simulink model "sdbe_8pac_11"  (R2012b)
settings: Solver=VariableStepDiscrete  SolverMode=SingleTasking  StartTime=0.0  StopTime=10000  RelTol=1e-3
PreLoadFcn:
  | counter_vals
undefined symbols (not defined in the file or in its folder): sfp
libraries: xbsIndex_r4 x9355, casper_library_misc x39, casper_library_delays x27, dspsigops x16, xps_library x10, r2dbe_vdif_lib x4, r2dbe_adc_lib x3, simulink x1
(part 31 of 79)

== system sdbe_8pac_11/valid_eof_snap_0x/bram ==
  addr : Inport
  data_in : Inport  Port=2
  we : Inport  Port=3
  calc_add : Subsystem  mask{data_width=16, addr_width=14, sample_rate=sample_rate}
      mask prompts: data_width "data width"; addr_width "address width"; sample_rate "sample rate"
  convert_addr : xbsIndex_r4/Convert  gui_display_data_type=Fixed-point  arith_type=Unsigned  n_bits=addr_width  bin_pt=0  float_type=Single  exp_bits=8  fraction_bits=24  quantization=Truncate  overflow=Wrap  en=off  latency=0  dbl_ovrd=off  pipeline=off  block_type=convert
      settings: xl_area=[0, 0, 0, 0, 0, 0, 0]
  convert_din1 : xbsIndex_r4/Convert  gui_display_data_type=Fixed-point  arith_type=Unsigned  n_bits=16  bin_pt=0  float_type=Single  exp_bits=8  fraction_bits=24  quantization=Truncate  overflow=Wrap  en=off  latency=0  dbl_ovrd=off  pipeline=off  block_type=convert
      settings: xl_area=[0, 0, 0, 0, 0, 0, 0]
  convert_we : xbsIndex_r4/Convert  gui_display_data_type=Fixed-point  arith_type=Unsigned  n_bits=1  bin_pt=0  float_type=Single  exp_bits=8  fraction_bits=24  quantization=Truncate  overflow=Wrap  en=off  latency=0  dbl_ovrd=off  pipeline=off  block_type=convert
      settings: xl_area=[0, 0, 0, 0, 0, 0, 0]
  mem : Subsystem
  munge_in : Subsystem  AncestorBlock=casper_library_flow_control/munge  mask(munge){divisions=1, div_size=16, order=[0], arith_type_out=Unsigned, bin_pt_out=0}
      mask prompts: divisions "Number of divisions"; div_size "Division size (bits)"; order "Division packing order"; arith_type_out "Output arithmetic type"; bin_pt_out "Output binary point"
      mask help: Splits an input bus into the specified number of divisions and then recombines them in the order specified (most significant division = 0,least = number divisions-1)
      mask init:
      | munge_init(gcb, ...
      |     'divisions', divisions, ...
      |     'div_size', div_size, ...
      |     'order', order, ...
      |     'arith_type_out', arith_type_out, ...
      |     'bin_pt_out', bin_pt_out);
      settings: AttributesFormatString=|
      | split:16
      | join:0
      | Unsigned [16,0]
      mask TypeOptions arith_type_out: Unsigned | Signed  (2's comp) | Floating-point
  munge_out : Subsystem  AncestorBlock=casper_library_flow_control/munge  mask(munge){divisions=1, div_size=16, order=[0], arith_type_out=Unsigned, bin_pt_out=0}
      mask prompts: divisions "Number of divisions"; div_size "Division size (bits)"; order "Division packing order"; arith_type_out "Output arithmetic type"; bin_pt_out "Output binary point"
      mask help: Splits an input bus into the specified number of divisions and then recombines them in the order specified (most significant division = 0,least = number divisions-1)
      mask init:
      | munge_init(gcb, ...
      |     'divisions', divisions, ...
      |     'div_size', div_size, ...
      |     'order', order, ...
      |     'arith_type_out', arith_type_out, ...
      |     'bin_pt_out', bin_pt_out);
      settings: AttributesFormatString=|
      | split:16
      | join:0
      | Unsigned [16,0]
      mask TypeOptions arith_type_out: Unsigned | Signed  (2's comp) | Floating-point
  sdbe_8pac_11_valid_eof_snap_0x_bram_addr : xbsIndex_r4/Gateway Out  inherit_from_input=off  hdl_port=on  timing_constraint=None  locs_specified=off  LOCs={'A5','B9','A9','C1','A3','G6','E9','A6','A7','A8','B8','B1','B3','D9','B5','B4','B6','C2'}  UseAsDAC=off  DACChannel='1'  block_type=gatewayout
      settings: infoedit="Gateway out block.  Converts Xilinx fixed point inputs into ouputs of type Simulink integer, double, or fixed point.<P><P>Hardware notes:  In hardware these blocks become top level output ports or are discarded, depending on how they are configured."  xl_area=[0, 0, 0, 0, 0, 0, 0]  sginterface={'Nallatech'=>{'xdspkit'=>{'non_memory_mapped_port'=>'uprev_Shared_BRAM_addr'}},'Xilinx'=>{'jtaghwcosim'=>{'non_memory_mapped_port'=>'uprev_Shared_BRAM_addr'},'xdspkit'=>{'non_memory_mapped_port'=>'uprev_Shared_BRAM_addr'}}}
  sdbe_8pac_11_valid_eof_snap_0x_bram_data_in : xbsIndex_r4/Gateway Out  inherit_from_input=off  hdl_port=on  timing_constraint=None  locs_specified=off  LOCs={'B21','B22','A22','B23','B19','C19','A20','A21','A23','B24','A24','A25','E18','D18','C18','B18'}  UseAsDAC=off  DACChannel='1'  block_type=gatewayout
      settings: infoedit="Gateway out block.  Converts Xilinx fixed point inputs into ouputs of type Simulink integer, double, or fixed point.<P><P>Hardware notes:  In hardware these blocks become top level output ports or are discarded, depending on how they are configured."  xl_area=[0, 0, 0, 0, 0, 0, 0]  sginterface={'Nallatech'=>{'xdspkit'=>{'non_memory_mapped_port'=>'uprev_Shared_BRAM_data_in'}},'Xilinx'=>{'jtaghwcosim'=>{'non_memory_mapped_port'=>'uprev_Shared_BRAM_data_in'},'xdspkit'=>{'non_memory_mapped_port'=>'uprev_Shared_BRAM_data_in'}}}
  sdbe_8pac_11_valid_eof_snap_0x_bram_data_out : xbsIndex_r4/Gateway In  gui_display_data_type=Fixed-point  arith_type=Unsigned  n_bits=16  bin_pt=0  preci_type=Single  exp_width=8  frac_width=24  quantization=Truncate  overflow=Wrap  period=sample_rate  dbl_ovrd=off  timing_constraint=None  locs_specified=off  LOCs={}  UseAsADC=off  ADCChannel='1'  inherit_from_input=off  hdl_port=on  block_type=gatewayin
      settings: xl_area=[0, 0, 0, 0, 0, 0, 0]
  sdbe_8pac_11_valid_eof_snap_0x_bram_we : xbsIndex_r4/Gateway Out  inherit_from_input=off  hdl_port=on  timing_constraint=None  locs_specified=off  LOCs={'A14'}  UseAsDAC=off  DACChannel='1'  block_type=gatewayout
      settings: infoedit="Gateway out block.  Converts Xilinx fixed point inputs into ouputs of type Simulink integer, double, or fixed point.<P><P>Hardware notes:  In hardware these blocks become top level output ports or are discarded, depending on how they are configured."  xl_area=[0, 0, 0, 0, 0, 0, 0]
  data_out : Outport
  wires:
  convert_addr/1 -> sdbe_8pac_11_valid_eof_snap_0x_bram_addr/1
  convert_din1/1 -> sdbe_8pac_11_valid_eof_snap_0x_bram_data_in/1
  data_in/1 -> munge_in/1(din)
  calc_add/1(out) -> convert_addr/1
  sdbe_8pac_11_valid_eof_snap_0x_bram_we/1 -> mem/3(In3)
  sdbe_8pac_11_valid_eof_snap_0x_bram_data_in/1 -> mem/2(In2)
  sdbe_8pac_11_valid_eof_snap_0x_bram_addr/1 -> mem/1(In1)
  convert_we/1 -> sdbe_8pac_11_valid_eof_snap_0x_bram_we/1
  sdbe_8pac_11_valid_eof_snap_0x_bram_data_out/1 -> munge_out/1(din)
  mem/1(Out1) -> sdbe_8pac_11_valid_eof_snap_0x_bram_data_out/1
  addr/1 -> calc_add/1(in)
  we/1 -> convert_we/1
  munge_out/1(dout) -> data_out/1
  munge_in/1(dout) -> convert_din1/1

== system sdbe_8pac_11/valid_eof_snap_0x/ctrl ==
  sim_1 : Inport
  io_delay : xbsIndex_r4/Delay  rst=off  infoeditControl=Selection of Reset will increase slice count due to use of real FFs and instead of SRLs  en=off  latency=0  dbl_ovrd=off  reg_retiming=on  block_type=delay
  reint1 : xbsIndex_r4/Reinterpret  force_arith_type=on  arith_type=Unsigned  force_bin_pt=on  bin_pt=0  block_type=reinterpret
  sdbe_8pac_11_valid_eof_snap_0x_ctrl_user_data_out : xbsIndex_r4/Gateway In  gui_display_data_type=Fixed-point  arith_type=Unsigned  n_bits=32  bin_pt=0  preci_type=Single  exp_width=8  frac_width=24  quantization="Round  (unbiased: +/- Inf)"  overflow=Saturate  period=1  dbl_ovrd=off  timing_constraint=None  locs_specified=off  LOCs={}  UseAsADC=off  ADCChannel='1'  inherit_from_input=off  hdl_port=on  block_type=gatewayin
  slice_reg : xbsIndex_r4/Slice  nbits=32  boolean_output=off  mode=Lower Bit Location + Width  bit1=0  base1=MSB of Input  bit0=0  base0=LSB of Input  dbl_ovrd=off  block_type=slice
  in_reg : Outport
  wires:
  sdbe_8pac_11_valid_eof_snap_0x_ctrl_user_data_out/1 -> io_delay/1
  sim_1/1 -> sdbe_8pac_11_valid_eof_snap_0x_ctrl_user_data_out/1
  io_delay/1 -> slice_reg/1
  slice_reg/1 -> reint1/1
  reint1/1 -> in_reg/1

== system sdbe_8pac_11/valid_eof_snap_0x/status ==
  out_reg : Inport
  assert_reg : xbsIndex_r4/Assert  assert_type=on  type_source=Explicitly  gui_display_data_type=Fixed-point  arith_type=Unsigned  n_bits=32  bin_pt=0  preci_type=Single  exp_width=8  frac_width=24  assert_rate=off  rate_source=Explicitly  period=1  output_port=on  block_type=assert
  cast_gw : xbsIndex_r4/Convert  gui_display_data_type=Fixed-point  arith_type=Unsigned  n_bits=32  bin_pt=0  float_type=Single  exp_bits=8  fraction_bits=24  quantization=Truncate  overflow=Wrap  en=off  latency=0  dbl_ovrd=off  pipeline=off  block_type=convert
  io_delay : xbsIndex_r4/Delay  rst=off  infoeditControl=Selection of Reset will increase slice count due to use of real FFs and instead of SRLs  en=off  latency=0  dbl_ovrd=off  reg_retiming=on  block_type=delay
  reint1 : xbsIndex_r4/Reinterpret  force_arith_type=on  arith_type=Unsigned  force_bin_pt=on  bin_pt=0  block_type=reinterpret
  sdbe_8pac_11_valid_eof_snap_0x_status_user_data_in : xbsIndex_r4/Gateway Out  inherit_from_input=off  hdl_port=on  timing_constraint=None  locs_specified=off  LOCs={}  UseAsDAC=off  DACChannel='1'  block_type=gatewayout
  sim_out : Outport
  wires:
  io_delay/1 -> cast_gw/1
  cast_gw/1 -> sdbe_8pac_11_valid_eof_snap_0x_status_user_data_in/1
  sdbe_8pac_11_valid_eof_snap_0x_status_user_data_in/1 -> sim_out/1
  out_reg/1 -> assert_reg/1
  assert_reg/1 -> reint1/1
  reint1/1 -> io_delay/1

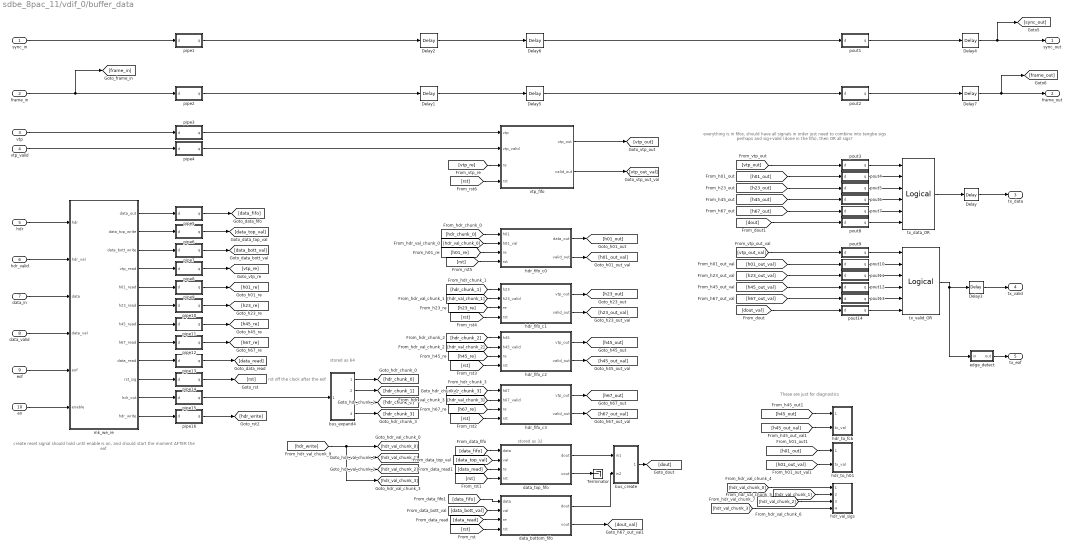
== system sdbe_8pac_11/vdif_0/buffer_data ==
  note: These are just for diagnostics
  note: rst off the clock after the eof
  note: create reset signal
      | should hold until enable is on, and should start the moment AFTER the eof
  note: everything is in fifos, should have all signals in order
      | just need to combine into tengbe sigs
      |
      | perhaps and sig+valid (done in the fifo), then OR all sigs?
  note: stored as 32
  note: stored as 64
  sync_in : Inport
  frame_in : Inport  Port=2
  vtp : Inport  Port=3
  vtp_valid : Inport  Port=4
  hdr : Inport  Port=5
  hdr_valid : Inport  Port=6
  data_in : Inport  Port=7
  data_valid : Inport  Port=8
  eof : Inport  Port=9
  en : Inport  Port=10
  Delay{,3..7} (6 alike) : xbsIndex_r4/Delay  rst=off  infoeditControl=Selection of Reset will increase slice count due to use of real FFs and instead of SRLs  en=off  latency=1  dbl_ovrd=off  reg_retiming=off  block_type=delay
  Delay1 : xbsIndex_r4/Delay  rst=off  infoeditControl=Selection of Reset will increase slice count due to use of real FFs and instead of SRLs  en=off  latency=128  dbl_ovrd=off  reg_retiming=off  block_type=delay
  Delay2 : xbsIndex_r4/Delay  rst=off  infoeditControl=Selection of Reset will increase slice count due to use of real FFs and instead of SRLs  en=off  latency=128  dbl_ovrd=off  reg_retiming=off  block_type=delay
  Terminator : Terminator
  bus_create : Subsystem  AncestorBlock=casper_library_flow_control/bus_create  mask(bus_create){inputNum=2}
      mask prompts: inputNum "Number of inputs:"
      mask init:
      | bus_create_init(gcb,...
      |     'inputNum', inputNum);
  bus_expand4 : Subsystem  AncestorBlock=casper_library_flow_control/bus_expand  mask(bus_expand){mode=divisions of equal size, outputNum=4, outputWidth=64, outputBinaryPt=0, outputArithmeticType=0, show_format=off, outputToWorkspace=off, variablePrefix=out, outputToModelAsWell=on}
      mask prompts: outputNum "Number of outputs:"; outputWidth "Output width:"; outputBinaryPt "Output binary point position:"; outputArithmeticType "Output arithmetic type (ufix=0, fix=1, bool=2):"; show_format "Print format string?"; outputToWorkspace "Output to workspace?"; variablePrefix "Variable name prefix:"; outputToModelAsWell "Output to model as well?"
      mask help:
      | Expands a 'bus' made using a bus_create or Xilinx
      | concat block.
      | The input will be divided into the specified number
      | of outputs with the specified arithmetic types.
      | Divisions are made from most significant bit.
      mask init: same as sdbe_8pac_11/get_data_from_pkt/scope/bus_expand1
      settings: AttributesFormatString=4 outputs
      mask TypeOptions mode: divisions of equal size | divisions of arbitrary size
      mask Callback mode: bus_expand_callback();
      mask Callback outputWidth: bus_expand_callback();
      mask Callback outputToWorkspace: bus_expand_callback();
  data_bottom_fifo : Subsystem
  data_top_fifo : Subsystem
  edge_detect : Subsystem  AncestorBlock=casper_library_misc/edge_detect  mask(edge_detect){edge=Falling, polarity=Active High, x_in=[0 0.08 0.08 0.16 0.16 0.24 0.24 0.32 0.32 0.4], y_in=[-1 -1  1  1  1  1  1  1  1  1], x_out=[0.6 0.68 0.68 0.76 0.76 0.84 0.84 0.92 0.92 1], y_out=[-1 -1  1  1 -1 -1 -1 -1 -1 -1]}
      mask prompts: edge "Edge Type"; polarity "Output Polarity"; x_in "Input X Positions"; y_in "Input Y Positions"; x_out "Output X Positions"; y_out "Output Y Positions"
      mask help: Output is active for one-cycle after each edge of the specified type (i.e. rising, falling or both).
      mask init: same as sdbe_8pac_11/vdif_0/edge_detect
      settings: AttributesFormatString=|
      | falling edges
      | active high
      mask Help: Output is active for one-cycle after each edge of the specified type (i.e. rising, falling, or both).  Latency is zero.
      mask TypeOptions edge: Rising | Falling | Both
      mask TypeOptions polarity: Active High | Active Low
      mask Display:
      | plot(x_in_num,0.5+y_in_num*0.2);
      | plot(x_out_num,0.5+y_out_num*0.2);
  hdr_fifo_c0 : Subsystem
  hdr_fifo_c1 : Subsystem
  hdr_fifo_c2 : Subsystem
  hdr_fifo_c3 : Subsystem
  hdr_to_fcb : Subsystem
  hdr_to_h01 : Subsystem
  hdr_val_sigs : Subsystem
  mk_we_re : Subsystem
  pipe1 : Subsystem  AncestorBlock=casper_library_delays/pipeline  mask(pipeline){latency=4}
      mask help:
      | An explicitly laid-out delay line to avoid mapping to SRL16s
      | for use in pipelining to help achieve timing closure.
      mask init:
      | pipeline_init(gcb,'latency',latency);
      settings: AttributesFormatString=Latency = %<latency>
      mask Display:
      | port_label('input', 1, 'd');
      | port_label('output', 1, 'q');
      | disp(['Z^-', num2str(latency)]);
  pipe10 : Subsystem  AncestorBlock=casper_library_delays/pipeline  mask(pipeline){latency=4}
      mask help:
      | An explicitly laid-out delay line to avoid mapping to SRL16s
      | for use in pipelining to help achieve timing closure.
      mask init:
      | pipeline_init(gcb,'latency',latency);
      settings: AttributesFormatString=Latency = %<latency>
      mask Display:
      | port_label('input', 1, 'd');
      | port_label('output', 1, 'q');
      | disp(['Z^-', num2str(latency)]);
  pipe11 : Subsystem  AncestorBlock=casper_library_delays/pipeline  mask(pipeline){latency=4}
      mask help:
      | An explicitly laid-out delay line to avoid mapping to SRL16s
      | for use in pipelining to help achieve timing closure.
      mask init:
      | pipeline_init(gcb,'latency',latency);
      settings: AttributesFormatString=Latency = %<latency>
      mask Display:
      | port_label('input', 1, 'd');
      | port_label('output', 1, 'q');
      | disp(['Z^-', num2str(latency)]);
  pipe12 : Subsystem  AncestorBlock=casper_library_delays/pipeline  mask(pipeline){latency=4}
      mask help:
      | An explicitly laid-out delay line to avoid mapping to SRL16s
      | for use in pipelining to help achieve timing closure.
      mask init:
      | pipeline_init(gcb,'latency',latency);
      settings: AttributesFormatString=Latency = %<latency>
      mask Display:
      | port_label('input', 1, 'd');
      | port_label('output', 1, 'q');
      | disp(['Z^-', num2str(latency)]);
  pipe13 : Subsystem  AncestorBlock=casper_library_delays/pipeline  mask(pipeline){latency=4}
      mask help:
      | An explicitly laid-out delay line to avoid mapping to SRL16s
      | for use in pipelining to help achieve timing closure.
      mask init:
      | pipeline_init(gcb,'latency',latency);
      settings: AttributesFormatString=Latency = %<latency>
      mask Display:
      | port_label('input', 1, 'd');
      | port_label('output', 1, 'q');
      | disp(['Z^-', num2str(latency)]);
  pipe14 : Subsystem  AncestorBlock=casper_library_delays/pipeline  mask(pipeline){latency=4}
      mask help:
      | An explicitly laid-out delay line to avoid mapping to SRL16s
      | for use in pipelining to help achieve timing closure.
      mask init:
      | pipeline_init(gcb,'latency',latency);
      settings: AttributesFormatString=Latency = %<latency>
      mask Display:
      | port_label('input', 1, 'd');
      | port_label('output', 1, 'q');
      | disp(['Z^-', num2str(latency)]);
  pipe15 : Subsystem  AncestorBlock=casper_library_delays/pipeline  mask(pipeline){latency=4}
      mask help:
      | An explicitly laid-out delay line to avoid mapping to SRL16s
      | for use in pipelining to help achieve timing closure.
      mask init:
      | pipeline_init(gcb,'latency',latency);
      settings: AttributesFormatString=Latency = %<latency>
      mask Display:
      | port_label('input', 1, 'd');
      | port_label('output', 1, 'q');
      | disp(['Z^-', num2str(latency)]);
  pipe16 : Subsystem  AncestorBlock=casper_library_delays/pipeline  mask(pipeline){latency=4}
      mask help:
      | An explicitly laid-out delay line to avoid mapping to SRL16s
      | for use in pipelining to help achieve timing closure.
      mask init:
      | pipeline_init(gcb,'latency',latency);
      settings: AttributesFormatString=Latency = %<latency>
      mask Display:
      | port_label('input', 1, 'd');
      | port_label('output', 1, 'q');
      | disp(['Z^-', num2str(latency)]);
  pipe2 : Subsystem  AncestorBlock=casper_library_delays/pipeline  mask(pipeline){latency=4}
      mask help:
      | An explicitly laid-out delay line to avoid mapping to SRL16s
      | for use in pipelining to help achieve timing closure.
      mask init:
      | pipeline_init(gcb,'latency',latency);
      settings: AttributesFormatString=Latency = %<latency>
      mask Display:
      | port_label('input', 1, 'd');
      | port_label('output', 1, 'q');
      | disp(['Z^-', num2str(latency)]);
  pipe3 : Subsystem  AncestorBlock=casper_library_delays/pipeline  mask(pipeline){latency=4}
      mask help:
      | An explicitly laid-out delay line to avoid mapping to SRL16s
      | for use in pipelining to help achieve timing closure.
      mask init:
      | pipeline_init(gcb,'latency',latency);
      settings: AttributesFormatString=Latency = %<latency>
      mask Display:
      | port_label('input', 1, 'd');
      | port_label('output', 1, 'q');
      | disp(['Z^-', num2str(latency)]);
  pipe4 : Subsystem  AncestorBlock=casper_library_delays/pipeline  mask(pipeline){latency=4}
      mask help:
      | An explicitly laid-out delay line to avoid mapping to SRL16s
      | for use in pipelining to help achieve timing closure.
      mask init:
      | pipeline_init(gcb,'latency',latency);
      settings: AttributesFormatString=Latency = %<latency>
      mask Display:
      | port_label('input', 1, 'd');
      | port_label('output', 1, 'q');
      | disp(['Z^-', num2str(latency)]);
  pipe5 : Subsystem  AncestorBlock=casper_library_delays/pipeline  mask(pipeline){latency=4}
      mask help:
      | An explicitly laid-out delay line to avoid mapping to SRL16s
      | for use in pipelining to help achieve timing closure.
      mask init:
      | pipeline_init(gcb,'latency',latency);
      settings: AttributesFormatString=Latency = %<latency>
      mask Display:
      | port_label('input', 1, 'd');
      | port_label('output', 1, 'q');
      | disp(['Z^-', num2str(latency)]);
  pipe6 : Subsystem  AncestorBlock=casper_library_delays/pipeline  mask(pipeline){latency=4}
      mask help:
      | An explicitly laid-out delay line to avoid mapping to SRL16s
      | for use in pipelining to help achieve timing closure.
      mask init:
      | pipeline_init(gcb,'latency',latency);
      settings: AttributesFormatString=Latency = %<latency>
      mask Display:
      | port_label('input', 1, 'd');
      | port_label('output', 1, 'q');
      | disp(['Z^-', num2str(latency)]);
  pipe7 : Subsystem  AncestorBlock=casper_library_delays/pipeline  mask(pipeline){latency=4}
      mask help:
      | An explicitly laid-out delay line to avoid mapping to SRL16s
      | for use in pipelining to help achieve timing closure.
      mask init:
      | pipeline_init(gcb,'latency',latency);
      settings: AttributesFormatString=Latency = %<latency>
      mask Display:
      | port_label('input', 1, 'd');
      | port_label('output', 1, 'q');
      | disp(['Z^-', num2str(latency)]);
  pipe8 : Subsystem  AncestorBlock=casper_library_delays/pipeline  mask(pipeline){latency=4}
      mask help:
      | An explicitly laid-out delay line to avoid mapping to SRL16s
      | for use in pipelining to help achieve timing closure.
      mask init:
      | pipeline_init(gcb,'latency',latency);
      settings: AttributesFormatString=Latency = %<latency>
      mask Display:
      | port_label('input', 1, 'd');
      | port_label('output', 1, 'q');
      | disp(['Z^-', num2str(latency)]);
  pipe9 : Subsystem  AncestorBlock=casper_library_delays/pipeline  mask(pipeline){latency=4}
      mask help:
      | An explicitly laid-out delay line to avoid mapping to SRL16s
      | for use in pipelining to help achieve timing closure.
      mask init:
      | pipeline_init(gcb,'latency',latency);
      settings: AttributesFormatString=Latency = %<latency>
      mask Display:
      | port_label('input', 1, 'd');
      | port_label('output', 1, 'q');
      | disp(['Z^-', num2str(latency)]);
  pout1 : Subsystem  AncestorBlock=casper_library_delays/pipeline  mask(pipeline){latency=3}
      mask help:
      | An explicitly laid-out delay line to avoid mapping to SRL16s
      | for use in pipelining to help achieve timing closure.
      mask init:
      | pipeline_init(gcb,'latency',latency);
      settings: AttributesFormatString=Latency = %<latency>
      mask Display:
      | port_label('input', 1, 'd');
      | port_label('output', 1, 'q');
      | disp(['Z^-', num2str(latency)]);
  pout10 : Subsystem  AncestorBlock=casper_library_delays/pipeline  mask(pipeline){latency=3}
      mask help:
      | An explicitly laid-out delay line to avoid mapping to SRL16s
      | for use in pipelining to help achieve timing closure.
      mask init:
      | pipeline_init(gcb,'latency',latency);
      settings: AttributesFormatString=Latency = %<latency>
      mask Display:
      | port_label('input', 1, 'd');
      | port_label('output', 1, 'q');
      | disp(['Z^-', num2str(latency)]);
  pout11 : Subsystem  AncestorBlock=casper_library_delays/pipeline  mask(pipeline){latency=3}
      mask help:
      | An explicitly laid-out delay line to avoid mapping to SRL16s
      | for use in pipelining to help achieve timing closure.
      mask init:
      | pipeline_init(gcb,'latency',latency);
      settings: AttributesFormatString=Latency = %<latency>
      mask Display:
      | port_label('input', 1, 'd');
      | port_label('output', 1, 'q');
      | disp(['Z^-', num2str(latency)]);
  pout12 : Subsystem  AncestorBlock=casper_library_delays/pipeline  mask(pipeline){latency=3}
      mask help:
      | An explicitly laid-out delay line to avoid mapping to SRL16s
      | for use in pipelining to help achieve timing closure.
      mask init:
      | pipeline_init(gcb,'latency',latency);
      settings: AttributesFormatString=Latency = %<latency>
      mask Display:
      | port_label('input', 1, 'd');
      | port_label('output', 1, 'q');
      | disp(['Z^-', num2str(latency)]);
  pout13 : Subsystem  AncestorBlock=casper_library_delays/pipeline  mask(pipeline){latency=3}
      mask help:
      | An explicitly laid-out delay line to avoid mapping to SRL16s
      | for use in pipelining to help achieve timing closure.
      mask init:
      | pipeline_init(gcb,'latency',latency);
      settings: AttributesFormatString=Latency = %<latency>
      mask Display:
      | port_label('input', 1, 'd');
      | port_label('output', 1, 'q');
      | disp(['Z^-', num2str(latency)]);
  pout14 : Subsystem  AncestorBlock=casper_library_delays/pipeline  mask(pipeline){latency=3}
      mask help:
      | An explicitly laid-out delay line to avoid mapping to SRL16s
      | for use in pipelining to help achieve timing closure.
      mask init:
      | pipeline_init(gcb,'latency',latency);
      settings: AttributesFormatString=Latency = %<latency>
      mask Display:
      | port_label('input', 1, 'd');
      | port_label('output', 1, 'q');
      | disp(['Z^-', num2str(latency)]);
  pout2 : Subsystem  AncestorBlock=casper_library_delays/pipeline  mask(pipeline){latency=3}
      mask help:
      | An explicitly laid-out delay line to avoid mapping to SRL16s
      | for use in pipelining to help achieve timing closure.
      mask init:
      | pipeline_init(gcb,'latency',latency);
      settings: AttributesFormatString=Latency = %<latency>
      mask Display:
      | port_label('input', 1, 'd');
      | port_label('output', 1, 'q');
      | disp(['Z^-', num2str(latency)]);
  pout3 : Subsystem  AncestorBlock=casper_library_delays/pipeline  mask(pipeline){latency=3}
      mask help:
      | An explicitly laid-out delay line to avoid mapping to SRL16s
      | for use in pipelining to help achieve timing closure.
      mask init:
      | pipeline_init(gcb,'latency',latency);
      settings: AttributesFormatString=Latency = %<latency>
      mask Display:
      | port_label('input', 1, 'd');
      | port_label('output', 1, 'q');
      | disp(['Z^-', num2str(latency)]);
  pout4 : Subsystem  AncestorBlock=casper_library_delays/pipeline  mask(pipeline){latency=3}
      mask help:
      | An explicitly laid-out delay line to avoid mapping to SRL16s
      | for use in pipelining to help achieve timing closure.
      mask init:
      | pipeline_init(gcb,'latency',latency);
      settings: AttributesFormatString=Latency = %<latency>
      mask Display:
      | port_label('input', 1, 'd');
      | port_label('output', 1, 'q');
      | disp(['Z^-', num2str(latency)]);
  pout5 : Subsystem  AncestorBlock=casper_library_delays/pipeline  mask(pipeline){latency=3}
      mask help:
      | An explicitly laid-out delay line to avoid mapping to SRL16s
      | for use in pipelining to help achieve timing closure.
      mask init:
      | pipeline_init(gcb,'latency',latency);
      settings: AttributesFormatString=Latency = %<latency>
      mask Display:
      | port_label('input', 1, 'd');
      | port_label('output', 1, 'q');
      | disp(['Z^-', num2str(latency)]);
  pout6 : Subsystem  AncestorBlock=casper_library_delays/pipeline  mask(pipeline){latency=3}
      mask help:
      | An explicitly laid-out delay line to avoid mapping to SRL16s
      | for use in pipelining to help achieve timing closure.
      mask init:
      | pipeline_init(gcb,'latency',latency);
      settings: AttributesFormatString=Latency = %<latency>
      mask Display:
      | port_label('input', 1, 'd');
      | port_label('output', 1, 'q');
      | disp(['Z^-', num2str(latency)]);
  pout7 : Subsystem  AncestorBlock=casper_library_delays/pipeline  mask(pipeline){latency=3}
      mask help:
      | An explicitly laid-out delay line to avoid mapping to SRL16s
      | for use in pipelining to help achieve timing closure.
      mask init:
      | pipeline_init(gcb,'latency',latency);
      settings: AttributesFormatString=Latency = %<latency>
      mask Display:
      | port_label('input', 1, 'd');
      | port_label('output', 1, 'q');
      | disp(['Z^-', num2str(latency)]);
  pout8 : Subsystem  AncestorBlock=casper_library_delays/pipeline  mask(pipeline){latency=3}
      mask help:
      | An explicitly laid-out delay line to avoid mapping to SRL16s
      | for use in pipelining to help achieve timing closure.
      mask init:
      | pipeline_init(gcb,'latency',latency);
      settings: AttributesFormatString=Latency = %<latency>
      mask Display:
      | port_label('input', 1, 'd');
      | port_label('output', 1, 'q');
      | disp(['Z^-', num2str(latency)]);
  pout9 : Subsystem  AncestorBlock=casper_library_delays/pipeline  mask(pipeline){latency=3}
      mask help:
      | An explicitly laid-out delay line to avoid mapping to SRL16s
      | for use in pipelining to help achieve timing closure.
      mask init:
      | pipeline_init(gcb,'latency',latency);
      settings: AttributesFormatString=Latency = %<latency>
      mask Display:
      | port_label('input', 1, 'd');
      | port_label('output', 1, 'q');
      | disp(['Z^-', num2str(latency)]);
  tx_data_OR : xbsIndex_r4/Logical  logical_function=OR  inputs=6  en=off  latency=0  precision=Full  arith_type=Unsigned  n_bits=16  bin_pt=0  align_bp=on  dbl_ovrd=off  block_type=logical
  tx_valid_OR : xbsIndex_r4/Logical  logical_function=OR  inputs=6  en=off  latency=0  precision=Full  arith_type=Unsigned  n_bits=16  bin_pt=0  align_bp=on  dbl_ovrd=off  block_type=logical
  vtp_fifo : Subsystem
  sync_out : Outport
  frame_out : Outport  Port=2
  tx_data : Outport  Port=3
  tx_valid : Outport  Port=4
  tx_eof : Outport  Port=5
  wires:
  frame_in/1 -> pipe2/1(d), [frame_in]
  Delay1/1 -> Delay5/1
  Delay2/1 -> Delay6/1
  bus_expand4/1(msb_out4) -> [hdr_chunk_0]
  bus_expand4/2(out3) -> [hdr_chunk_1]
  bus_expand4/3(out2) -> [hdr_chunk_2]
  bus_expand4/4(lsb_out1) -> [hdr_chunk_3]
  [hdr_write] -> [hdr_val_chunk_2], [hdr_val_chunk_3], [hdr_val_chunk_1], [hdr_val_chunk_0]
  vtp_fifo/1(vtp_out) -> [vtp_out]
  vtp_fifo/2(valid_out) -> [vtp_out_val]
  [hdr_chunk_0] -> hdr_fifo_c0/1(h01)
  [hdr_val_chunk_0] -> hdr_fifo_c0/2(h01_val)
  [hdr_chunk_1] -> hdr_fifo_c1/1(h23)
  [hdr_val_chunk_1] -> hdr_fifo_c1/2(h23_valid)
  [hdr_chunk_2] -> hdr_fifo_c2/1(h45)
  [hdr_val_chunk_2] -> hdr_fifo_c2/2(h45_valid)
  [hdr_chunk_3] -> hdr_fifo_c3/1(h67)
  [hdr_val_chunk_3] -> hdr_fifo_c3/2(h67_valid)
  [h67_re] -> hdr_fifo_c3/3(re)
  [h45_re] -> hdr_fifo_c2/3(re)
  [h23_re] -> hdr_fifo_c1/3(re)
  [h01_re] -> hdr_fifo_c0/3(re)
  [vtp_re] -> vtp_fifo/3(re)
  [data_bott_val] -> data_bottom_fifo/2(val)
  [data_read] -> data_bottom_fifo/3(re)
  [data_read] -> data_top_fifo/3(re)
  [data_top_val] -> data_top_fifo/2(val)
  [data_fifo] -> data_top_fifo/1(data)
  [data_fifo] -> data_bottom_fifo/1(data)
  data_top_fifo/1(dout) -> bus_create/1(in1)
  data_bottom_fifo/1(dout) -> bus_create/2(in2)
  [rst] -> data_bottom_fifo/4(rst)
  [rst] -> data_top_fifo/4(rst)
  [rst] -> hdr_fifo_c3/4(rst)
  [rst] -> hdr_fifo_c2/4(rst)
  [rst] -> hdr_fifo_c1/4(rst)
  [rst] -> hdr_fifo_c0/4(rst)
  [rst] -> vtp_fifo/4(rst)
  hdr_fifo_c0/1(data_out) -> [h01_out]
  hdr_fifo_c0/2(valid_out) -> [h01_out_val]
  hdr_fifo_c1/1(vtp_out) -> [h23_out]
  hdr_fifo_c1/2(valid_out) -> [h23_out_val]
  hdr_fifo_c2/1(vtp_out) -> [h45_out]
  hdr_fifo_c2/2(valid_out) -> [h45_out_val]
  hdr_fifo_c3/1(vtp_out) -> [h67_out]
  hdr_fifo_c3/2(valid_out) -> [h67_out_val]
  data_bottom_fifo/2(vout) -> [dout_val]
  data_top_fifo/2(vout) -> Terminator/1
  bus_create/1(bus_out) -> [dout]
  edge_detect/1(out) -> tx_eof/1
  tx_data_OR/1 -> Delay/1
  Delay/1 -> tx_data/1
  tx_valid_OR/1 -> edge_detect/1(in), Delay3/1
  Delay3/1 -> tx_valid/1
  Delay4/1 -> [sync_out], sync_out/1
  Delay7/1 -> frame_out/1, [frame_out]
  [h45_out] -> hdr_to_fcb/1(tx_data)
  [h45_out_val] -> hdr_to_fcb/2(tx_val)
  [h01_out] -> hdr_to_h01/1(tx_data)
  [h01_out_val] -> hdr_to_h01/2(tx_val)
  [hdr_val_chunk_0] -> hdr_val_sigs/1(hdr_val)
  [hdr_val_chunk_1] -> hdr_val_sigs/2(hdr_val1)
  [hdr_val_chunk_2] -> hdr_val_sigs/3(hdr_val2)
  [hdr_val_chunk_3] -> hdr_val_sigs/4(hdr_val3)
  hdr/1 -> mk_we_re/1(hdr)
  hdr_valid/1 -> mk_we_re/2(hdr_val)
  data_in/1 -> mk_we_re/3(data)
  data_valid/1 -> mk_we_re/4(data_val)
  eof/1 -> mk_we_re/5(eof)
  en/1 -> mk_we_re/6(enable)
  sync_in/1 -> pipe1/1(d)
  pipe1/1(q) -> Delay2/1
  mk_we_re/9(data_read) -> pipe13/1(d)
  mk_we_re/5(h01_read) -> pipe9/1(d)
  mk_we_re/2(data_top_write) -> pipe6/1(d)
  mk_we_re/8(h67_read) -> pipe12/1(d)
  mk_we_re/7(h45_read) -> pipe11/1(d)
  mk_we_re/10(rst_sig) -> pipe14/1(d)
  mk_we_re/11(hdr_out) -> pipe15/1(d)
  mk_we_re/6(h23_read) -> pipe10/1(d)
  mk_we_re/3(data_bott_write) -> pipe7/1(d)
  mk_we_re/12(hdr_write) -> pipe16/1(d)
  mk_we_re/1(data_out) -> pipe5/1(d)
  mk_we_re/4(vtp_read) -> pipe8/1(d)
  pipe5/1(q) -> [data_fifo]
  pipe6/1(q) -> [data_top_val]
  pipe7/1(q) -> [data_bott_val]
  pipe8/1(q) -> [vtp_re]
  pipe9/1(q) -> [h01_re]
  pipe10/1(q) -> [h23_re]
  pipe11/1(q) -> [h45_re]
  pipe12/1(q) -> [h67_re]
  pipe13/1(q) -> [data_read]
  pipe14/1(q) -> [rst]
  pipe15/1(q) -> bus_expand4/1(bus_in)
  pipe16/1(q) -> [hdr_write]
  vtp/1 -> pipe3/1(d)
  vtp_valid/1 -> pipe4/1(d)
  pipe4/1(q) -> vtp_fifo/2(vtp_valid)
  pipe3/1(q) -> vtp_fifo/1(vtp)
  pipe2/1(q) -> Delay1/1
  Delay6/1 -> pout1/1(d)
  pout1/1(q) -> Delay4/1
  pout11/1(q) -> tx_valid_OR/3
  pout10/1(q) -> tx_valid_OR/2
  pout9/1(q) -> tx_valid_OR/1
  pout12/1(q) -> tx_valid_OR/4
  pout13/1(q) -> tx_valid_OR/5
  pout14/1(q) -> tx_valid_OR/6
  pout5/1(q) -> tx_data_OR/3
  pout3/1(q) -> tx_data_OR/1
  pout8/1(q) -> tx_data_OR/6
  pout7/1(q) -> tx_data_OR/5
  pout4/1(q) -> tx_data_OR/2
  pout6/1(q) -> tx_data_OR/4
  [vtp_out] -> pout3/1(d)
  [h01_out] -> pout4/1(d)
  [h23_out] -> pout5/1(d)
  [h45_out] -> pout6/1(d)
  [h67_out] -> pout7/1(d)
  [dout] -> pout8/1(d)
  [vtp_out_val] -> pout9/1(d)
  [h01_out_val] -> pout10/1(d)
  [h23_out_val] -> pout11/1(d)
  [h45_out_val] -> pout12/1(d)
  [h67_out_val] -> pout13/1(d)
  [dout_val] -> pout14/1(d)
  Delay5/1 -> pout2/1(d)
  pout2/1(q) -> Delay7/1

== system sdbe_8pac_11/vdif_0/edge_detect ==
  in : Inport
  Delay : xbsIndex_r4/Delay  rst=off  infoeditControl=Selection of Reset will increase slice count due to use of real FFs and instead of SRLs  en=off  latency=1  dbl_ovrd=off  reg_retiming=off  block_type=delay
      settings: xl_area=[0, 0, 0, 0, 0, 0, 0]
  Inverter : xbsIndex_r4/Inverter  en=off  latency=0  dbl_ovrd=off  block_type=inv
      settings: xl_area=[0, 0, 0, 0, 0, 0, 0]
  edge_op : xbsIndex_r4/Logical  logical_function=AND  inputs=2  en=off  latency=0  precision=Full  arith_type=Unsigned  n_bits=8  bin_pt=2  align_bp=on  dbl_ovrd=off  block_type=logical
      settings: xl_area=[0, 0, 0, 0, 0, 0, 0]
  out : Outport
  wires:
  Inverter/1 -> edge_op/1
  edge_op/1 -> out/1
  in/1 -> Inverter/1, Delay/1
  Delay/1 -> edge_op/2

== system sdbe_8pac_11/vdif_0/enable ==
  sim_1 : Inport
  io_delay : xbsIndex_r4/Delay  rst=off  infoeditControl=Selection of Reset will increase slice count due to use of real FFs and instead of SRLs  en=off  latency=0  dbl_ovrd=off  reg_retiming=on  block_type=delay
  reint1 : xbsIndex_r4/Reinterpret  force_arith_type=on  arith_type=Unsigned  force_bin_pt=on  bin_pt=0  block_type=reinterpret
  sdbe_8pac_11_vdif_0_enable_user_data_out : xbsIndex_r4/Gateway In  gui_display_data_type=Fixed-point  arith_type=Unsigned  n_bits=32  bin_pt=0  preci_type=Single  exp_width=8  frac_width=24  quantization="Round  (unbiased: +/- Inf)"  overflow=Saturate  period=1  dbl_ovrd=off  timing_constraint=None  locs_specified=off  LOCs={}  UseAsADC=off  ADCChannel='1'  inherit_from_input=off  hdl_port=on  block_type=gatewayin
  slice_reg : xbsIndex_r4/Slice  nbits=32  boolean_output=off  mode=Lower Bit Location + Width  bit1=0  base1=MSB of Input  bit0=0  base0=LSB of Input  dbl_ovrd=off  block_type=slice
  in_reg : Outport
  wires:
  sdbe_8pac_11_vdif_0_enable_user_data_out/1 -> io_delay/1
  sim_1/1 -> sdbe_8pac_11_vdif_0_enable_user_data_out/1
  io_delay/1 -> slice_reg/1
  slice_reg/1 -> reint1/1
  reint1/1 -> in_reg/1

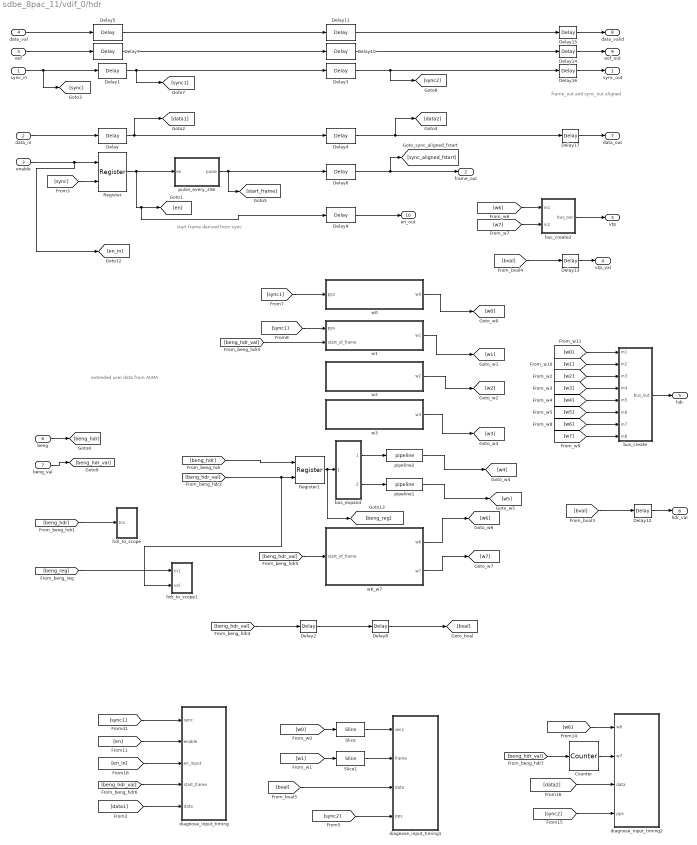
== system sdbe_8pac_11/vdif_0/hdr ==
  note: frame_out and sync_out aligned
  note: start frame derived from sync
  note: extended user data
      | from ALMA
  sync_in : Inport
  data_in : Inport  Port=2
  enable : Inport  Port=3
  data_val : Inport  Port=4
  eof : Inport  Port=5
  beng : Inport  Port=6
  beng_val : Inport  Port=7
  Counter : xbsIndex_r4/Counter  cnt_type=Free Running  cnt_to=Inf  operation=Up  start_count=2^32-1  cnt_by_val=1  arith_type=Unsigned  n_bits=32  bin_pt=0  load_pin=off  rst=off  en=on  explicit_period=on  period=1  dbl_ovrd=off  use_behavioral_HDL=off  implementation=Fabric  block_type=counter
  Delay{,1..11} (12 alike) : xbsIndex_r4/Delay  rst=off  infoeditControl=Selection of Reset will increase slice count due to use of real FFs and instead of SRLs  en=off  latency=1  dbl_ovrd=off  reg_retiming=off  block_type=delay
  Delay{12..17} (6 alike) : xbsIndex_r4/Delay  rst=off  infoeditControl=Selection of Reset will increase slice count due to use of real FFs and instead of SRLs  en=off  latency=2  dbl_ovrd=off  reg_retiming=off  block_type=delay
  Register : xbsIndex_r4/Register  init=0  rst=off  en=on  dbl_ovrd=off  block_type=register
  Register1 : xbsIndex_r4/Register  init=0  rst=off  en=on  dbl_ovrd=off  block_type=register
  Slice : xbsIndex_r4/Slice  nbits=30  boolean_output=off  mode=Lower Bit Location + Width  bit1=0  base1=MSB of Input  bit0=0  base0=LSB of Input  dbl_ovrd=off  block_type=slice
  Slice1 : xbsIndex_r4/Slice  nbits=24  boolean_output=off  mode=Lower Bit Location + Width  bit1=0  base1=MSB of Input  bit0=0  base0=LSB of Input  dbl_ovrd=off  block_type=slice
  bus_create : Subsystem  AncestorBlock=casper_library_flow_control/bus_create  mask(bus_create){inputNum=8}
      mask prompts: inputNum "Number of inputs:"
      mask init:
      | bus_create_init(gcb,...
      |     'inputNum', inputNum);
  bus_create2 : Subsystem  AncestorBlock=casper_library_flow_control/bus_create  mask(bus_create){inputNum=2}
      mask prompts: inputNum "Number of inputs:"
      mask init:
      | bus_create_init(gcb,...
      |     'inputNum', inputNum);
  bus_expand : Subsystem  AncestorBlock=casper_library_flow_control/bus_expand  mask(bus_expand){mode=divisions of equal size, outputNum=2, outputWidth=32, outputBinaryPt=0, outputArithmeticType=0, show_format=off, outputToWorkspace=off, variablePrefix=out, outputToModelAsWell=on}
      mask prompts: outputNum "Number of outputs:"; outputWidth "Output width:"; outputBinaryPt "Output binary point position:"; outputArithmeticType "Output arithmetic type (ufix=0, fix=1, bool=2):"; show_format "Print format string?"; outputToWorkspace "Output to workspace?"; variablePrefix "Variable name prefix:"; outputToModelAsWell "Output to model as well?"
      mask help:
      | Expands a 'bus' made using a bus_create or Xilinx
      | concat block.
      | The input will be divided into the specified number
      | of outputs with the specified arithmetic types.
      | Divisions are made from most significant bit.
      mask init: same as sdbe_8pac_11/get_data_from_pkt/scope/bus_expand1
      settings: AttributesFormatString=2 outputs
      mask TypeOptions mode: divisions of equal size | divisions of arbitrary size
      mask Callback mode: bus_expand_callback();
      mask Callback outputWidth: bus_expand_callback();
      mask Callback outputToWorkspace: bus_expand_callback();
  diagnose_input_timing : Subsystem
  diagnose_input_timing1 : Subsystem
  diagnose_input_timing2 : Subsystem
  hdr_to_scope : Subsystem
  hdr_to_scope1 : Subsystem
  pipeline1 : casper_library_delays/pipeline  latency=1
      settings: AttributesFormatString=Latency = %<latency>
  pipeline2 : casper_library_delays/pipeline  latency=1
      settings: AttributesFormatString=Latency = %<latency>
  pulse_every_256 : Subsystem  mask{per=256}
      mask prompts: per "period"
      mask help: Creates a pulse duration 1 with period from 2 to <large number>. Pulse begins with enable signal, no latency.
  w0 : Subsystem
  w1 : Subsystem
  w2 : Subsystem
  w3 : Subsystem
  w6_w7 : Subsystem
  sync_out : Outport
  frame_out : Outport  Port=2
  vtp : Outport  Port=3
  vtp_val : Outport  Port=4
  hdr : Outport  Port=5
  hdr_val : Outport  Port=6
  data_out : Outport  Port=7
  data_valid : Outport  Port=8
  eof_out : Outport  Port=9
  en_out : Outport  Port=10
  wires:
  bus_expand/1(msb_out2) -> pipeline2/1
  [en] -> diagnose_input_timing/2(enable)
  [sync1] -> diagnose_input_timing/1(sync)
  [beng_hdr_val] -> w1/2(start_of_frame)
  [sync1] -> w1/1(pps)
  [sync1] -> w0/1(pps)
  sync_in/1 -> [sync], Delay1/1
  data_in/1 -> Delay/1
  w0/1(w0) -> [w0]
  w1/1(w1) -> [w1]
  w2/1(w2) -> [w2]
  w3/1(w3) -> [w3]
  pipeline2/1 -> [w4]
  w6_w7/1(w6) -> [w6]
  w6_w7/2(w7) -> [w7]
  [beng_hdr_val] -> w6_w7/1(start_of_frame)
  enable/1 -> [en_in], Register/1
  [sync] -> Register/2
  Slice1/1 -> diagnose_input_timing1/2(frame)
  Slice/1 -> diagnose_input_timing1/1(secs)
  [bval] -> diagnose_input_timing1/3(data)
  [sync2] -> diagnose_input_timing1/4(pps)
  Delay/1 -> Delay4/1, [data1]
  Delay1/1 -> Delay3/1, [sync1]
  [w0] -> Slice/1
  [w1] -> Slice1/1
  pulse_every_256/1(pulse) -> Delay6/1, [start_frame]
  Counter/1 -> diagnose_input_timing2/2(w7)
  [w6] -> diagnose_input_timing2/1(w6)
  [data2] -> diagnose_input_timing2/3(data)
  [sync2] -> diagnose_input_timing2/4(pps)
  [w6] -> bus_create2/1(in1)
  [w7] -> bus_create2/2(in2)
  [en_in] -> diagnose_input_timing/3(en_input)
  [beng_hdr_val] -> diagnose_input_timing/4(start_frame)
  [data1] -> diagnose_input_timing/5(data)
  pipeline1/1 -> [w5]
  [beng_hdr] -> Register1/1
  bus_expand/2(lsb_out1) -> pipeline1/1
  Register1/1 -> [beng_reg], bus_expand/1(bus_in)
  [beng_hdr_val] -> hdr_to_scope1/2(val), Register1/2
  [beng_hdr] -> hdr_to_scope/1(In1)
  [beng_reg] -> hdr_to_scope1/1(In1)
  data_val/1 -> Delay5/1
  Delay5/1 -> Delay11/1
  [beng_hdr_val] -> Counter/1
  [w1] -> bus_create/2(in2)
  [w2] -> bus_create/3(in3)
  [w0] -> bus_create/1(in1)
  [w3] -> bus_create/4(in4)
  [w4] -> bus_create/5(in5)
  [w5] -> bus_create/6(in6)
  [w6] -> bus_create/7(in7)
  [w7] -> bus_create/8(in8)
  [beng_hdr_val] -> Delay2/1
  bus_create2/1(bus_out) -> vtp/1
  [bval] -> Delay13/1
  bus_create/1(bus_out) -> hdr/1
  [bval] -> Delay12/1
  eof/1 -> Delay7/1
  Delay7/1 -> Delay10/1
  Register/1 -> Delay9/1, [en], pulse_every_256/1(en)
  beng/1 -> [beng_hdr]
  beng_val/1 -> [beng_hdr_val]
  Delay2/1 -> Delay8/1
  Delay3/1 -> [sync2], Delay16/1
  Delay4/1 -> Delay17/1, [data2]
  Delay6/1 -> [sync_aligned_fstart], frame_out/1
  Delay9/1 -> en_out/1
  Delay10/1 -> Delay14/1
  Delay11/1 -> Delay15/1
  Delay8/1 -> [bval]
  Delay12/1 -> hdr_val/1
  Delay13/1 -> vtp_val/1
  Delay14/1 -> eof_out/1
  Delay15/1 -> data_valid/1
  Delay16/1 -> sync_out/1
  Delay17/1 -> data_out/1

== system sdbe_8pac_11/vdif_0/hdr_to_scope1 ==
  note: VTP so need to wait one more clock
  tx_data : Inport
  tx_val : Inport  Port=2
  tx_eof : Inport  Port=3
  Disregard Subsystem : xbsIndex_r4/Disregard Subsystem  Tag=discardX  block_type=disregard
  Gateway Out1 : xbsIndex_r4/Gateway Out  inherit_from_input=off  hdl_port=on  timing_constraint=None  locs_specified=off  LOCs={}  UseAsDAC=off  DACChannel='1'  block_type=gatewayout
  Gateway Out3 : xbsIndex_r4/Gateway Out  inherit_from_input=off  hdl_port=on  timing_constraint=None  locs_specified=off  LOCs={}  UseAsDAC=off  DACChannel='1'  block_type=gatewayout
  Gateway Out4 : xbsIndex_r4/Gateway Out  inherit_from_input=off  hdl_port=on  timing_constraint=None  locs_specified=off  LOCs={}  UseAsDAC=off  DACChannel='1'  block_type=gatewayout
  Mux1 : Mux  Inputs=2
  diagnose_beng_hdr : Subsystem
  wires:
  Gateway Out4/1 -> Mux1/2
  Gateway Out3/1 -> Mux1/1
  tx_data/1 -> Gateway Out1/1  "_yellow__b_pink__f_blue"
  Mux1/1 -> diagnose_beng_hdr/2(tx_val)  "val_sigs"
  Gateway Out1/1 -> diagnose_beng_hdr/1(tx_data)  "data"
  tx_val/1 -> Gateway Out3/1
  tx_eof/1 -> Gateway Out4/1

== system sdbe_8pac_11/vdif_0/hdr_to_scope3 ==
  tx_data : Inport
  tx_val : Inport  Port=2
  Delay : xbsIndex_r4/Delay  rst=off  infoeditControl=Selection of Reset will increase slice count due to use of real FFs and instead of SRLs  en=off  latency=3  dbl_ovrd=off  reg_retiming=off  block_type=delay
  Delay1 : xbsIndex_r4/Delay  rst=off  infoeditControl=Selection of Reset will increase slice count due to use of real FFs and instead of SRLs  en=off  latency=2  dbl_ovrd=off  reg_retiming=off  block_type=delay
  Delay2 : xbsIndex_r4/Delay  rst=off  infoeditControl=Selection of Reset will increase slice count due to use of real FFs and instead of SRLs  en=off  latency=4  dbl_ovrd=off  reg_retiming=off  block_type=delay
  Delay3 : xbsIndex_r4/Delay  rst=off  infoeditControl=Selection of Reset will increase slice count due to use of real FFs and instead of SRLs  en=off  latency=1  dbl_ovrd=off  reg_retiming=off  block_type=delay
  Delay4 : xbsIndex_r4/Delay  rst=off  infoeditControl=Selection of Reset will increase slice count due to use of real FFs and instead of SRLs  en=off  latency=4  dbl_ovrd=off  reg_retiming=off  block_type=delay
  Slice1 : xbsIndex_r4/Slice  nbits=64  boolean_output=off  mode=Upper Bit Location + Width  bit1=0  base1=MSB of Input  bit0=0  base0=LSB of Input  dbl_ovrd=off  block_type=slice
  Slice2 : xbsIndex_r4/Slice  nbits=64  boolean_output=off  mode=Upper Bit Location + Width  bit1=0  base1=MSB of Input  bit0=0  base0=LSB of Input  dbl_ovrd=off  block_type=slice
  Slice4 : xbsIndex_r4/Slice  nbits=64  boolean_output=off  mode=Upper Bit Location + Width  bit1=0  base1=MSB of Input  bit0=0  base0=LSB of Input  dbl_ovrd=off  block_type=slice
  beng_w45 : Subsystem
  data_p0r : Subsystem
  posedge{,1..4} (5 alike) : casper_library_misc/posedge  Tag=Rising Edge Detector
  pulse_ext : casper_library_misc/pulse_ext  pulse_len=128
  vtp : Subsystem
  w01 : Subsystem
  w23 : Subsystem
  w67 : Subsystem
  wires:
  posedge/1 -> Delay/1
  Slice4/1 -> beng_w45/1(data)
  Delay/1 -> beng_w45/3(spec_val)
  posedge1/1 -> Delay3/1
  tx_data/1 -> Slice2/1, data_p0r/1(data), w67/1(data), Slice1/1, w01/1(data), Slice4/1
  posedge2/1 -> Delay1/1
  Slice1/1 -> w23/1(data)
  Delay1/1 -> w23/3(spec_val)
  posedge3/1 -> vtp/3(spec_val)
  tx_val/1 -> vtp/2(val), w01/2(val), posedge1/1, posedge2/1, Delay4/1, data_p0r/2(val), w67/2(val), posedge4/1, w23/2(val), beng_w45/2(val), posedge3/1, posedge/1
  Slice2/1 -> vtp/1(data)
  posedge4/1 -> Delay2/1
  Delay2/1 -> w67/3(spec_val)
  Delay3/1 -> w01/3(spec_val)
  Delay4/1 -> pulse_ext/1
  pulse_ext/1 -> data_p0r/3(spec_val)

== system sdbe_8pac_11/vdif_0/little_end ==
  sim_1 : Inport
  io_delay : xbsIndex_r4/Delay  rst=off  infoeditControl=Selection of Reset will increase slice count due to use of real FFs and instead of SRLs  en=off  latency=0  dbl_ovrd=off  reg_retiming=on  block_type=delay
  reint1 : xbsIndex_r4/Reinterpret  force_arith_type=on  arith_type=Unsigned  force_bin_pt=on  bin_pt=0  block_type=reinterpret
  sdbe_8pac_11_vdif_0_little_end_user_data_out : xbsIndex_r4/Gateway In  gui_display_data_type=Fixed-point  arith_type=Unsigned  n_bits=32  bin_pt=0  preci_type=Single  exp_width=8  frac_width=24  quantization="Round  (unbiased: +/- Inf)"  overflow=Saturate  period=1  dbl_ovrd=off  timing_constraint=None  locs_specified=off  LOCs={}  UseAsADC=off  ADCChannel='1'  inherit_from_input=off  hdl_port=on  block_type=gatewayin
  slice_reg : xbsIndex_r4/Slice  nbits=32  boolean_output=off  mode=Lower Bit Location + Width  bit1=0  base1=MSB of Input  bit0=0  base0=LSB of Input  dbl_ovrd=off  block_type=slice
  in_reg : Outport
  wires:
  sdbe_8pac_11_vdif_0_little_end_user_data_out/1 -> io_delay/1
  sim_1/1 -> sdbe_8pac_11_vdif_0_little_end_user_data_out/1
  io_delay/1 -> slice_reg/1
  slice_reg/1 -> reint1/1
  reint1/1 -> in_reg/1

== system sdbe_8pac_11/vdif_0/pipeline1 ==
  d : Inport
  Register0 : xbsIndex_r4/Register  init=0  rst=off  en=off  dbl_ovrd=off  block_type=register
      settings: block_version=11.4
  q : Outport
  wires:
  d/1 -> Register0/1
  Register0/1 -> q/1

== system sdbe_8pac_11/vdif_0/pipeline2 ==
  d : Inport
  Register0 : xbsIndex_r4/Register  init=0  rst=off  en=off  dbl_ovrd=off  block_type=register
      settings: block_version=11.4
  q : Outport
  wires:
  d/1 -> Register0/1
  Register0/1 -> q/1

== system sdbe_8pac_11/vdif_0/pipeline4 ==
  d : Inport
  Register0 : xbsIndex_r4/Register  init=0  rst=off  en=off  dbl_ovrd=off  block_type=register
      settings: block_version=11.4
  q : Outport
  wires:
  d/1 -> Register0/1
  Register0/1 -> q/1

== system sdbe_8pac_11/vdif_0/pipeline6 ==
  d : Inport
  Register0 : xbsIndex_r4/Register  init=0  rst=off  en=off  dbl_ovrd=off  block_type=register
      settings: block_version=11.4
  q : Outport
  wires:
  d/1 -> Register0/1
  Register0/1 -> q/1

== system sdbe_8pac_11/vdif_0/reorder ==
  d_native : Inport
  Concat : xbsIndex_r4/Concat  num_inputs=16  dbl_ovrd=off  block_type=concat
  Subsystem : Subsystem
  d_ordered : Outport
  wires:
  Concat/1 -> d_ordered/1
  d_native/1 -> Subsystem/1(bus_in)
  Subsystem/1(msb_out16) -> Concat/16
  Subsystem/2(out15) -> Concat/15
  Subsystem/3(out14) -> Concat/14
  Subsystem/4(out13) -> Concat/13
  Subsystem/5(out12) -> Concat/12
  Subsystem/6(out11) -> Concat/11
  Subsystem/7(out10) -> Concat/10
  Subsystem/8(out9) -> Concat/9
  Subsystem/9(out8) -> Concat/8
  Subsystem/10(out7) -> Concat/7
  Subsystem/11(out6) -> Concat/6
  Subsystem/12(out5) -> Concat/5
  Subsystem/13(out4) -> Concat/4
  Subsystem/14(out3) -> Concat/3
  Subsystem/15(out2) -> Concat/2
  Subsystem/16(lsb_out1) -> Concat/1
